simulink model "ATABEY_sistem_modeli"  (R2025b)
settings: Solver=VariableStepAuto  StartTime=0.0  StopTime=simTime  RelTol=1e-3
undefined symbols (not defined in the file): u1max, u1min, u2max, u2min, u3max, u3min, u4max, u4min, x0
settings Model: Creator=erayacikgz  LastModifiedBy=erayacikgz

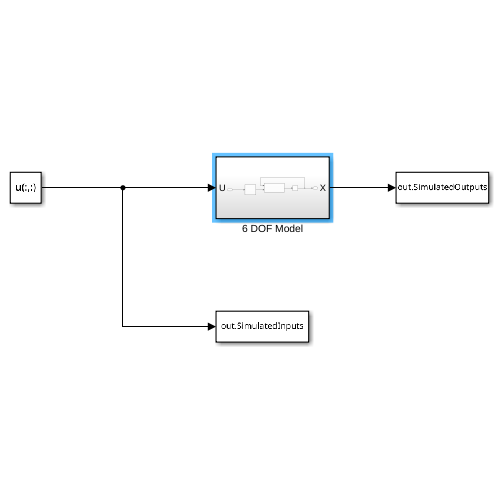
[thumbnail: Simulink's stored preview of the top-level diagram]
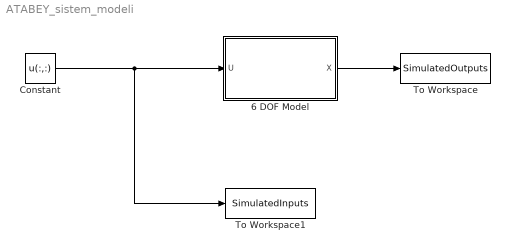
== system ATABEY_sistem_modeli ==
  6 DOF Model : Subsystem
  Constant : Constant  Value=u(:,:)
  To Workspace : ToWorkspace  VariableName=SimulatedOutputs  SaveFormat=Timeseries  SampleTime=-1
  To Workspace1 : ToWorkspace  VariableName=SimulatedInputs  SaveFormat=Timeseries  SampleTime=-1
  wires:
  6 DOF Model/1(X) -> To Workspace/1
  Constant/1 -> To Workspace1/1, 6 DOF Model/1(U)

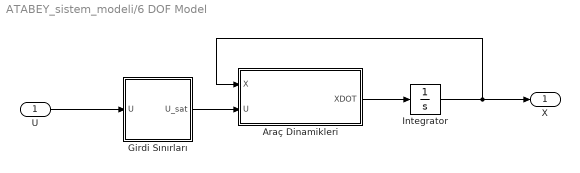
== system ATABEY_sistem_modeli/6 DOF Model ==
  U : Inport
  Araç Dinamikleri : MATLAB Function  TreatAsAtomicUnit=on
  Girdi Sınırları : Subsystem
  Integrator : Integrator  InitialCondition=x0
  X : Outport
  wires:
  Araç Dinamikleri/1(XDOT) -> Integrator/1
  Integrator/1 -> Araç Dinamikleri/1(X), X/1
  U/1 -> Girdi Sınırları/1(U)
  Girdi Sınırları/1(U_sat) -> Araç Dinamikleri/2(U)

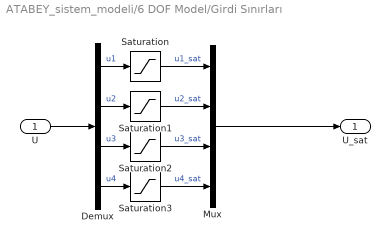
== system ATABEY_sistem_modeli/6 DOF Model/Girdi Sınırları ==
  U : Inport
  Demux : Demux
  Mux : Mux
  Saturation : Saturate  UpperLimit=u1max  LowerLimit=u1min
  Saturation1 : Saturate  UpperLimit=u2max  LowerLimit=u2min
  Saturation2 : Saturate  UpperLimit=u3max  LowerLimit=u3min
  Saturation3 : Saturate  UpperLimit=u4max  LowerLimit=u4min
  U_sat : Outport
  wires:
  Saturation2/1 -> Mux/3  "u3_sat"
  Mux/1 -> U_sat/1
  Demux/2 -> Saturation1/1  "u2"
  Demux/4 -> Saturation3/1  "u4"
  Saturation1/1 -> Mux/2  "u2_sat"
  Saturation/1 -> Mux/1  "u1_sat"
  Saturation3/1 -> Mux/4  "u4_sat"
  Demux/3 -> Saturation2/1  "u3"
  U/1 -> Demux/1
  Demux/1 -> Saturation/1  "u1"

== matlab function ATABEY_sistem_modeli/6 DOF Model/Araç Dinamikleri ==
  data: X input; U input; XDOT output
function XDOT   = ATABEY_model(X, U)

    [XDOT] = ATABEY_model(X, U);

end
